simulink model "ThirdTask"  (R2023b)
settings: Solver=ode23t  StartTime=0.0  StopTime=20  FixedStep=1e-4  RelTol=1e-3
libraries: slpidlib x2
settings Model: Creator=ycheb  LastModifiedBy=ycheb

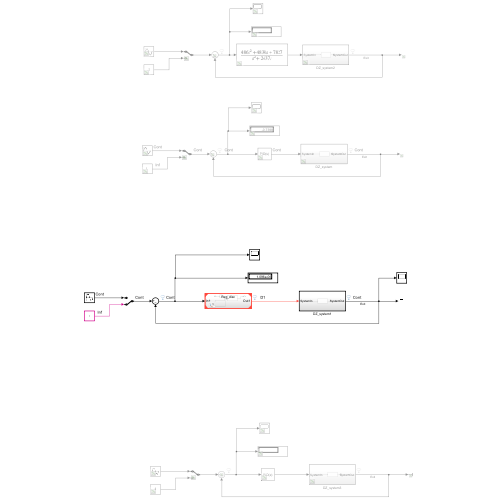
[thumbnail: Simulink's stored preview of the top-level diagram]
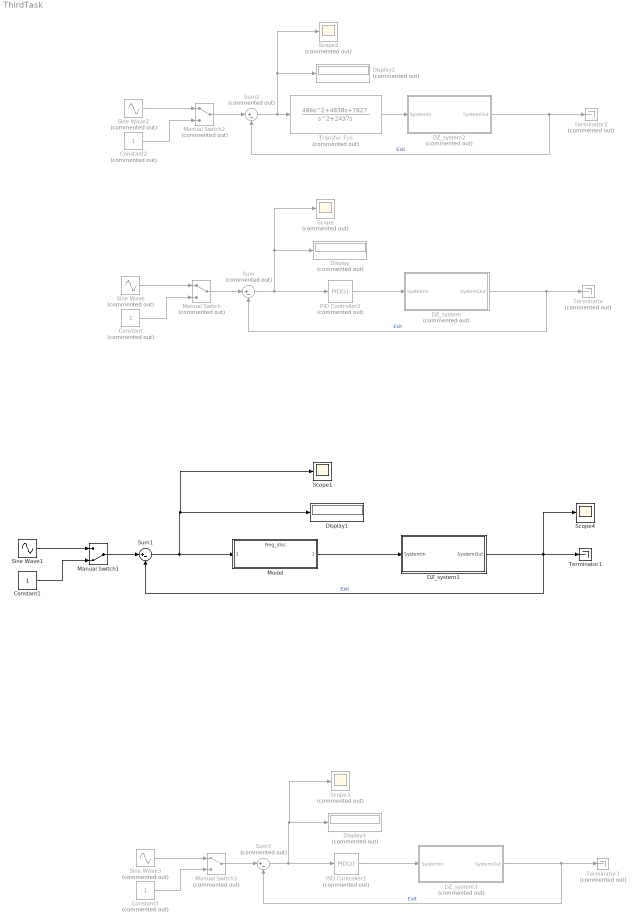
== system ThirdTask ==
  Constant : Constant  Commented=on
  Constant1 : Constant
  Constant2 : Constant  Commented=on
  Constant3 : Constant  Commented=on
  DZ_system : Subsystem  Commented=on
  DZ_system1 : Subsystem
  DZ_system2 : Subsystem  Commented=on
  DZ_system3 : Subsystem  Commented=on
  Display : Display  Commented=on
  Display1 : Display
  Display2 : Display  Commented=on
  Display3 : Display  Commented=on
  Manual Switch : ManualSwitch  Commented=on
  Manual Switch1 : ManualSwitch  CurrentSetting=0
  Manual Switch2 : ManualSwitch  Commented=on
  Manual Switch3 : ManualSwitch  Commented=on
  Model : ModelReference  ModelNameDialog=Reg_disc.slx  SimulationMode=Normal  ModelReferenceVersion=1.19
  PID Controller1 : slpidlib/PID Controller  Commented=on  Controller=PID  Form=Parallel  TimeDomain=Discrete-time  UseExternalTs=off  SampleTime=1e-4  IntegratorMethod=Forward Euler  FilterMethod=Forward Euler  ControllerParametersSource=internal  P=1.98391542251931  I=3.21168879545358  UseKiTs=off  D=0.198597393319278  N=2437.04094665053  UseFilter=on  TunerSelectOption=Transfer Function Based (PID Tuner App)  InitialConditionSource=internal  InitialConditionForIntegrator=0  InitialConditionForFilter=0  DifferentiatorICPrevScaledInput=0  ExternalReset=none  TrackingMode=off  Kt=1  LimitOutput=off  SatLimitsSource=internal  UpperSaturationLimit=inf  LowerSaturationLimit=-inf  LinearizeAsGain=on  AntiWindupMode=none  Kb=1  LimitIntegrator=off  UpperIntegratorSaturationLimit=inf  LowerIntegratorSaturationLimit=-inf  POutMin=[]  POutMax=[]  IOutMin=[]  IOutMax=[]  DOutMin=[]  DOutMax=[]  NOutMin=[]  NOutMax=[]  SumOutMin=[]  SumOutMax=[]  SaturationOutMin=[]  SaturationOutMax=[]  PParamMin=[]  PParamMax=[]  IParamMin=[]  IParamMax=[]  DParamMin=[]  DParamMax=[]  NParamMin=[]  NParamMax=[]  KbParamMin=[]  KbParamMax=[]  KtParamMin=[]  KtParamMax=[]  KbOutMin=[]  KbOutMax=[]  KtOutMin=[]  KtOutMax=[]  IntegratorOutMin=[]  IntegratorOutMax=[]  FilterOutMin=[]  FilterOutMax=[]  SumI1OutMin=[]  SumI1OutMax=[]  SumI2OutMin=[]  SumI2OutMax=[]  SumI3OutMin=[]  SumI3OutMax=[]  SumI4OutMin=[]  SumI4OutMax=[]  SumDOutMin=[]  SumDOutMax=[]  DifferentiatorOutMin=[]  DifferentiatorOutMax=[]  FilterDiffOutCoefMin=[]  FilterDiffOutCoefMax=[]  ReciprocalOutMin=[]  ReciprocalOutMax=[]  SumDenOutMin=[]  SumDenOutMax=[]  SumNumOutMin=[]  SumNumOutMax=[]  DivideOutMin=[]  DivideOutMax=[]  UdiffTsProdOutMin=[]  UdiffTsProdOutMax=[]  NTsProdOutMin=[]  NTsProdOutMax=[]  UintegralTsProdOutMin=[]  UintegralTsProdOutMax=[]  UngainTsProdOutMin=[]  UngainTsProdOutMax=[]  ClampingZeroOutDataTypeStr=Inherit: Inherit via back propagation  ClampingZeroOutMin=[]  ClampingZeroOutMax=[]  FilterDenConstantOutDataTypeStr=Inherit: Inherit via back propagation  FilterDenConstantOutMin=[]  FilterDenConstantOutMax=[]  PCopyOutDataTypeStr=Inherit: Inherit via back propagation  PCopyOutMin=[]  PCopyOutMax=[]  NCopyOutDataTypeStr=Inherit: Inherit via back propagation  NCopyOutMin=[]  NCopyOutMax=[]  IntegratorContinuousStateAttributes=''  IntegratorStateMustResolveToSignalObject=off  IntegratorRTWStateStorageClass=Auto  FilterContinuousStateAttributes=''  FilterStateMustResolveToSignalObject=off  FilterRTWStateStorageClass=Auto  ParallelPVariant=InternalParameters  IdealPVariant=Disabled  IVariant=InternalParameters  DVariant=InternalParameters  IntegratorVariant=Discrete  SatVariant=Disabled  AWVariant=Passthrough  PCopyVariant=Disabled  TRVariant=Disabled  FdbkBlocksVariant=Forward  IdealPFdbkVariant=Disabled  SatFdbkVariant=Disabled  DerivativeFilterVariant=ForwardEulerFilter  NVariant=InternalParameters  NCopyVariant=Disabled  FilterICVariant=InternalICsFilter  IntegratorICVariant=InternalICs  ExternalResetVariant=Disabled  TRSumVariant=Passthrough  SumFdbkVariant=Disabled  SumVariant=Sum_PID  TsampFilterVariant=InternalTs  TsampNgainVariant=Passthrough  TsampIntegralVariant=Disabled_SignalSpec  ExternalSaturationOutDataTypeStr=Inherit: Same as second input
  PID Controller2 : slpidlib/PID Controller  Commented=on  Controller=PID  Form=Parallel  TimeDomain=Continuous-time  UseExternalTs=off  SampleTime=-1  IntegratorMethod=Forward Euler  FilterMethod=Forward Euler  ControllerParametersSource=internal  P=1.72626593892633  I=0.624359128150613  UseKiTs=off  D=1.06047859947846  N=7085.10834495725  UseFilter=on  TunerSelectOption=Transfer Function Based (PID Tuner App)  InitialConditionSource=internal  InitialConditionForIntegrator=0  InitialConditionForFilter=0  DifferentiatorICPrevScaledInput=0  ExternalReset=none  TrackingMode=off  Kt=1  LimitOutput=off  SatLimitsSource=internal  UpperSaturationLimit=inf  LowerSaturationLimit=-inf  LinearizeAsGain=on  AntiWindupMode=none  Kb=1  LimitIntegrator=off  UpperIntegratorSaturationLimit=inf  LowerIntegratorSaturationLimit=-inf  POutMin=[]  POutMax=[]  IOutMin=[]  IOutMax=[]  DOutMin=[]  DOutMax=[]  NOutMin=[]  NOutMax=[]  SumOutMin=[]  SumOutMax=[]  SaturationOutMin=[]  SaturationOutMax=[]  PParamMin=[]  PParamMax=[]  IParamMin=[]  IParamMax=[]  DParamMin=[]  DParamMax=[]  NParamMin=[]  NParamMax=[]  KbParamMin=[]  KbParamMax=[]  KtParamMin=[]  KtParamMax=[]  KbOutMin=[]  KbOutMax=[]  KtOutMin=[]  KtOutMax=[]  IntegratorOutMin=[]  IntegratorOutMax=[]  FilterOutMin=[]  FilterOutMax=[]  SumI1OutMin=[]  SumI1OutMax=[]  SumI2OutMin=[]  SumI2OutMax=[]  SumI3OutMin=[]  SumI3OutMax=[]  SumI4OutMin=[]  SumI4OutMax=[]  SumDOutMin=[]  SumDOutMax=[]  DifferentiatorOutMin=[]  DifferentiatorOutMax=[]  FilterDiffOutCoefMin=[]  FilterDiffOutCoefMax=[]  ReciprocalOutMin=[]  ReciprocalOutMax=[]  SumDenOutMin=[]  SumDenOutMax=[]  SumNumOutMin=[]  SumNumOutMax=[]  DivideOutMin=[]  DivideOutMax=[]  UdiffTsProdOutMin=[]  UdiffTsProdOutMax=[]  NTsProdOutMin=[]  NTsProdOutMax=[]  UintegralTsProdOutMin=[]  UintegralTsProdOutMax=[]  UngainTsProdOutMin=[]  UngainTsProdOutMax=[]  ClampingZeroOutDataTypeStr=Inherit: Inherit via back propagation  ClampingZeroOutMin=[]  ClampingZeroOutMax=[]  FilterDenConstantOutDataTypeStr=Inherit: Inherit via back propagation  FilterDenConstantOutMin=[]  FilterDenConstantOutMax=[]  PCopyOutDataTypeStr=Inherit: Inherit via back propagation  PCopyOutMin=[]  PCopyOutMax=[]  NCopyOutDataTypeStr=Inherit: Inherit via back propagation  NCopyOutMin=[]  NCopyOutMax=[]  IntegratorContinuousStateAttributes=''  IntegratorStateMustResolveToSignalObject=off  IntegratorRTWStateStorageClass=Auto  FilterContinuousStateAttributes=''  FilterStateMustResolveToSignalObject=off  FilterRTWStateStorageClass=Auto  ParallelPVariant=InternalParameters  IdealPVariant=Disabled  IVariant=InternalParameters  DVariant=InternalParameters  IntegratorVariant=Continuous  SatVariant=Disabled  AWVariant=Passthrough  PCopyVariant=Disabled  TRVariant=Disabled  FdbkBlocksVariant=Forward  IdealPFdbkVariant=Disabled  SatFdbkVariant=Disabled  DerivativeFilterVariant=ContFilter  NVariant=InternalParameters  NCopyVariant=Disabled  FilterICVariant=InternalICsFilter  IntegratorICVariant=InternalICs  ExternalResetVariant=Disabled  TRSumVariant=Passthrough  SumFdbkVariant=Disabled  SumVariant=Sum_PID  TsampFilterVariant=InternalTs  TsampNgainVariant=Passthrough  TsampIntegralVariant=Disabled_SignalSpec  ExternalSaturationOutDataTypeStr=Inherit: Same as second input
  Scope : Scope  Commented=on
  Scope1 : Scope
  Scope2 : Scope  Commented=on
  Scope3 : Scope  Commented=on
  Scope4 : Scope
  Sine Wave : Sin  Commented=on  Amplitude=50  Frequency=0.5  SampleTime=0
  Sine Wave1 : Sin  Amplitude=50  Frequency=0.5  SampleTime=0
  Sine Wave2 : Sin  Commented=on  Amplitude=50  Frequency=0.5  SampleTime=0
  Sine Wave3 : Sin  Commented=on  Amplitude=50  Frequency=0.5  SampleTime=0
  Sum : Sum  Commented=on  Inputs=|+-
  Sum1 : Sum  Inputs=|+-
  Sum2 : Sum  Commented=on  Inputs=|+-
  Sum3 : Sum  Commented=on  Inputs=|+-
  Terminator : Terminator  Commented=on
  Terminator1 : Terminator
  Terminator2 : Terminator  Commented=on
  Terminator3 : Terminator  Commented=on
  Transfer Fcn : TransferFcn  Commented=on  Numerator=[486 4838 7827]  Denominator=[1 2437 0]
  wires:
  PID Controller2/1 -> DZ_system/1(SystemIn)
  DZ_system/1(SystemOut) -> Terminator/1, Sum/2  "Exit"
  Sine Wave/1 -> Manual Switch/1
  Constant/1 -> Manual Switch/2
  Manual Switch/1 -> Sum/1
  Sum/1 -> PID Controller2/1, Scope/1, Display/1
  Constant1/1 -> Manual Switch1/2
  Sine Wave1/1 -> Manual Switch1/1
  Manual Switch1/1 -> Sum1/1
  DZ_system1/1(SystemOut) -> Scope4/1, Terminator1/1, Sum1/2  "Exit"
  Sum1/1 -> Model/1, Scope1/1, Display1/1
  Manual Switch2/1 -> Sum2/1
  Sine Wave2/1 -> Manual Switch2/1
  DZ_system2/1(SystemOut) -> Terminator2/1, Sum2/2  "Exit"
  Constant2/1 -> Manual Switch2/2
  Sum2/1 -> Scope2/1, Display2/1, Transfer Fcn/1
  Transfer Fcn/1 -> DZ_system2/1(SystemIn)
  Sine Wave3/1 -> Manual Switch3/1
  DZ_system3/1(SystemOut) -> Terminator3/1, Sum3/2  "Exit"
  Manual Switch3/1 -> Sum3/1
  Sum3/1 -> PID Controller1/1, Scope3/1, Display3/1
  Constant3/1 -> Manual Switch3/2
  PID Controller1/1 -> DZ_system3/1(SystemIn)
  Model/1 -> DZ_system1/1(SystemIn)

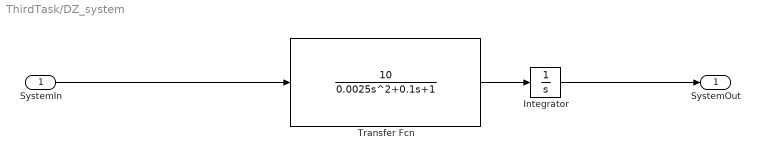
== system ThirdTask/DZ_system ==
  SystemIn : Inport
  Integrator : Integrator
  Transfer Fcn : TransferFcn  Numerator=[10]  Denominator=[0.0025 0.1 1]
  SystemOut : Outport
  wires:
  Transfer Fcn/1 -> Integrator/1
  Integrator/1 -> SystemOut/1
  SystemIn/1 -> Transfer Fcn/1

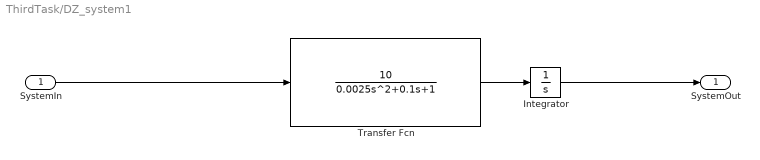
== system ThirdTask/DZ_system1 ==
  SystemIn : Inport
  Integrator : Integrator
  Transfer Fcn : TransferFcn  Numerator=[10]  Denominator=[0.0025 0.1 1]
  SystemOut : Outport
  wires:
  Transfer Fcn/1 -> Integrator/1
  Integrator/1 -> SystemOut/1
  SystemIn/1 -> Transfer Fcn/1

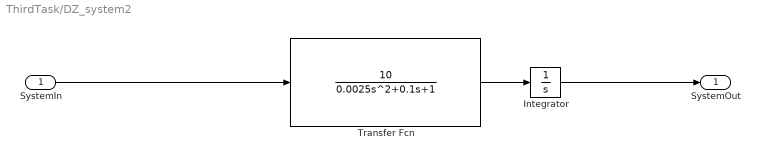
== system ThirdTask/DZ_system2 ==
  SystemIn : Inport
  Integrator : Integrator
  Transfer Fcn : TransferFcn  Numerator=[10]  Denominator=[0.0025 0.1 1]
  SystemOut : Outport
  wires:
  Transfer Fcn/1 -> Integrator/1
  Integrator/1 -> SystemOut/1
  SystemIn/1 -> Transfer Fcn/1

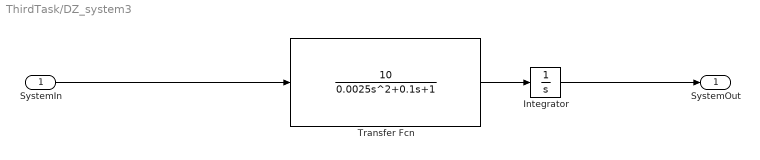
== system ThirdTask/DZ_system3 ==
  SystemIn : Inport
  Integrator : Integrator
  Transfer Fcn : TransferFcn  Numerator=[10]  Denominator=[0.0025 0.1 1]
  SystemOut : Outport
  wires:
  Transfer Fcn/1 -> Integrator/1
  Integrator/1 -> SystemOut/1
  SystemIn/1 -> Transfer Fcn/1
